simulink model "Feedback_System_Non_linear"  (R2024a)
settings: Solver=VariableStepAuto  StartTime=0.0  StopTime=10.0  RelTol=1e-3
values from neighbouring files (symbols this model uses):
  J = (m/12)*(l^2*cos(beta)^2+d^2*sin(beta)^2+w^2)    [Group10_Final_Code_Summer.m]    (also in Group10_Final_Main_Code_Winter.m)
  Kd = 5    [Group10_Final_Code_Summer.m]    (also in Group10_Final_Main_Code_Winter.m)
  Kf = 0.07    [Group10_Final_Code_Summer.m]    (also in Group10_Final_Main_Code_Winter.m)
  Kg = 3000    [Group10_Final_Code_Summer.m]    (also in Group10_Final_Main_Code_Winter.m)
  Kp = 0.318    [Group10_Final_Code_Summer.m]    (also in Group10_Final_Main_Code_Winter.m)
  Kt = 0.07    [Group10_Final_Code_Summer.m]    (also in Group10_Final_Main_Code_Winter.m)
  L = 1e-5    (= 1e-05)    [Group10_Final_Code_Summer.m]    (also in Group10_Final_Main_Code_Winter.m)
  R = 10    [Group10_Final_Code_Summer.m]    (also in Group10_Final_Main_Code_Winter.m)
settings Model: Creator=marin  LastModifiedBy=marin

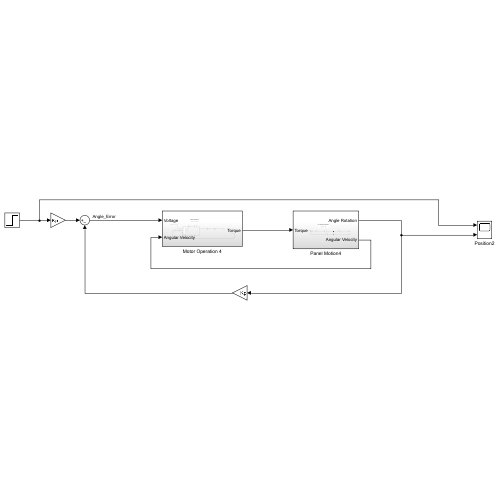
[thumbnail: Simulink's stored preview of the top-level diagram]
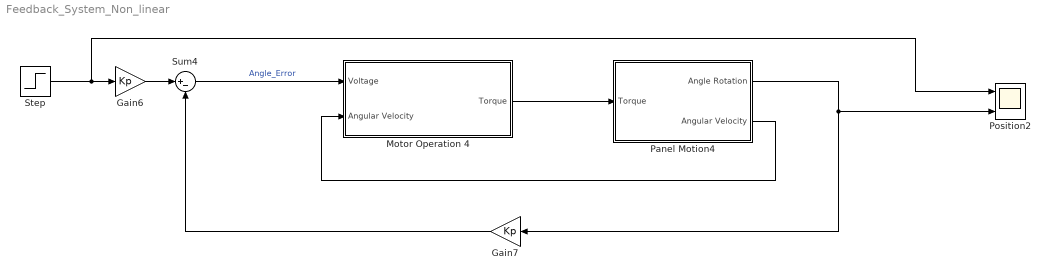
== system Feedback_System_Non_linear ==
  Gain6 : Gain  Gain=Kp
  Gain7 : Gain  Gain=Kp
  Motor Operation 4 : Subsystem
  Panel Motion4 : Subsystem
  Position2 : Scope  NumInputPorts=2
  Step : Step  SampleTime=0
  Sum4 : Sum  Inputs=|+-
  wires:
  Step/1 -> Gain6/1, Position2/1
  Gain6/1 -> Sum4/1
  Motor Operation 4/1(Torque) -> Panel Motion4/1(Torque)
  Panel Motion4/1(Angle Rotation) -> Position2/2, Gain7/1
  Sum4/1 -> Motor Operation 4/1(Voltage)  "Angle_Error"
  Gain7/1 -> Sum4/2
  Panel Motion4/2(Angular Velocity) -> Motor Operation 4/2(Angular Velocity)

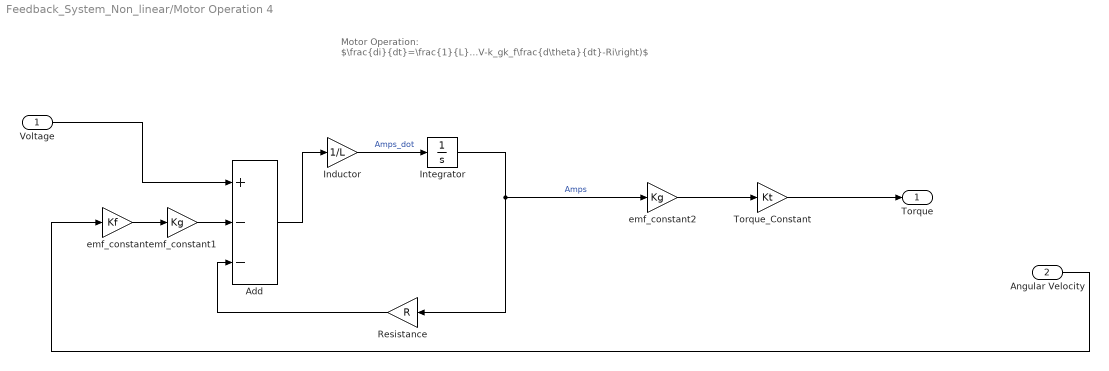
== system Feedback_System_Non_linear/Motor Operation 4 ==
  note: Motor Operation:
      | $\frac{di}{dt}=\frac{1}{L}\left(V-k_gk_f\frac{d\theta}{dt}-Ri\right)$
  Voltage : Inport
  Angular Velocity : Inport  Port=2
  Add : Sum  Inputs=+--
  Inductor : Gain  Gain=1/L
  Integrator : Integrator
  Resistance : Gain  Gain=R
  Torque_Constant : Gain  Gain=Kt
  emf_constant : Gain  Gain=Kf
  emf_constant1 : Gain  Gain=Kg
  emf_constant2 : Gain  Gain=Kg
  Torque : Outport
  wires:
  emf_constant2/1 -> Torque_Constant/1
  emf_constant1/1 -> Add/2
  Torque_Constant/1 -> Torque/1
  Integrator/1 -> emf_constant2/1, Resistance/1  "Amps"
  Voltage/1 -> Add/1
  Angular Velocity/1 -> emf_constant/1
  Inductor/1 -> Integrator/1  "Amps_dot"
  Add/1 -> Inductor/1
  Resistance/1 -> Add/3
  emf_constant/1 -> emf_constant1/1

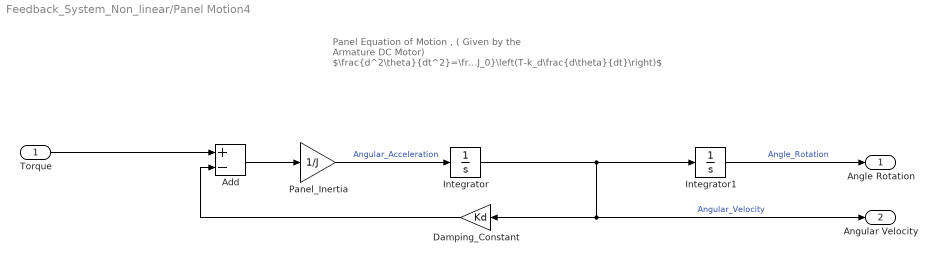
== system Feedback_System_Non_linear/Panel Motion4 ==
  note: Panel Equation of Motion ,
      | ( Given by the Armature DC Motor)
      | $\frac{d^2\theta}{dt^2}=\frac{1}{J_0}\left(T-k_d\frac{d\theta}{dt}\right)$
  Torque : Inport
  Add : Sum  Inputs=+-
  Damping_Constant : Gain  Gain=Kd
  Integrator : Integrator
  Integrator1 : Integrator
  Panel_Inertia : Gain  Gain=1/J
  Angle Rotation : Outport
  Angular Velocity : Outport  Port=2
  wires:
  Torque/1 -> Add/1
  Integrator/1 -> Integrator1/1, Damping_Constant/1, Angular Velocity/1  "Angular_Velocity"
  Damping_Constant/1 -> Add/2
  Add/1 -> Panel_Inertia/1
  Panel_Inertia/1 -> Integrator/1  "Angular_Acceleration"
  Integrator1/1 -> Angle Rotation/1  "Angle_Rotation"
